simulink model "arduino_serial_sendreceive"  (R2018a)
settings: Solver=FixedStepAuto  StartTime=0.0  StopTime=inf  FixedStep=0.005  RelTol=1e-3  EnableMultiTasking=on
undefined symbols (not defined in the file or in its folder): maxPWM, minPWM
libraries: arduinolib x3, simulink x1
settings Model: SimulationMode=external  ExtModeTrigDuration=2  Creator=The MathWorks, Inc.  LastModifiedBy=adiravishankara
settings SolverCC: AutoInsertRateTranBlk=on
settings OptimizationCC: PassReuseOutputArgsThreshold=0  MaxStackSize=64
settings DebuggingCC: ParameterTunabilityLossMsg=error
settings HardwareCC: ProdBitPerPointer=32  ProdBitPerSizeT=32  ProdBitPerPtrDiffT=32  ProdLargestAtomicInteger=Long  ProdLargestAtomicFloat=Double  ProdWordSize=32  ProdHWDeviceType=ARM Compatible->ARM Cortex  UseEmbeddedCoderFeatures=off
settings SFSimCC: MATLABDynamicMemAlloc=off
settings RTWCC: SystemTargetFile=ert.tlc  HardwareBoard=Arduino Due  TLCOptions=-aInlineSetEventsForThisBaseRateFcn=TLC_FALSE -aSuppressMultiTaskScheduler=TLC_FALSE -aRateBasedStepFcn=1  TemplateMakefile=ert_default_tmf  GenerateReport=on  Toolchain=Arduino ARM  BuildConfiguration=Faster Runs  LaunchReport=on
settings CodeAppCC: ForceParamTrailComments=on  OperatorAnnotations=on
settings ERTTargetCC: ERTCustomFileBanners=off  SupportContinuousTime=on  SupportNonInlinedSFcns=on  RemoveResetFunc=off  SupportVariableSizeSignals=on  ModelStepFunctionPrototypeControlCompliant=off

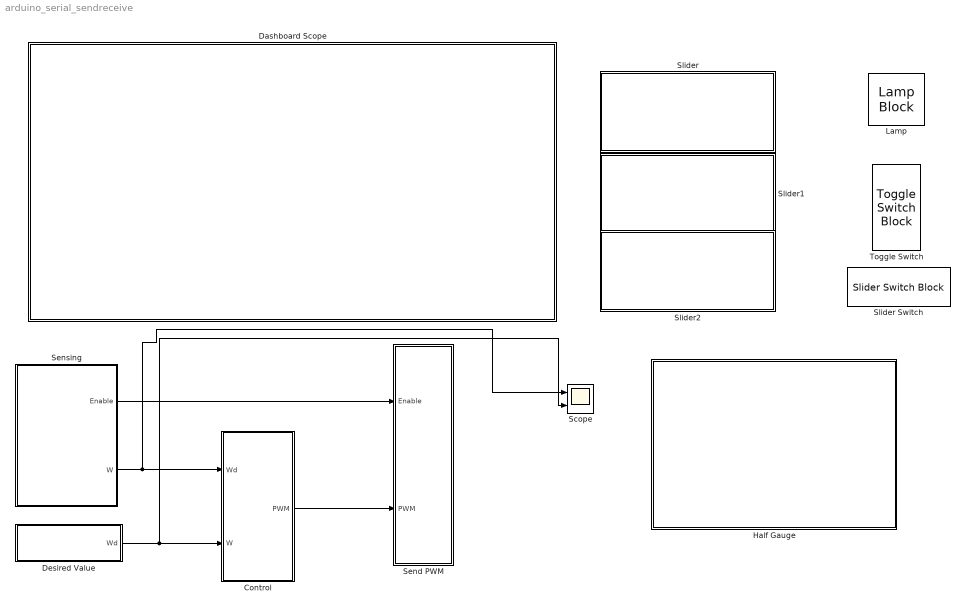
== system arduino_serial_sendreceive ==
  Control : Subsystem
  Dashboard Scope : Subsystem  DialogController=hmiCreateDDGDialog  IsWebBlock=on  mask(MWDashboardBlock){webBlockId=9cdac41f-9582-470c-8574-661c351767b2, webBlockType=sdiscope, ShowInitialText=on, HMISrcModelName=arduino_serial_sendreceive}
      mask prompts: webBlockId "WebBlock Id"; webBlockType "WebBlock Type"; HMISrcModelName "Source Model"
      mask help: SimulinkHMI:dialogs:HMIScopeDialogDesc
      mask Help: helpview([docroot '/mapfiles/simulink.map'], 'hmi_scope')
      mask Display:
      | if strcmp(get_param(bdroot(gcb),'BlockDiagramType'), 'library')
      |     image([(matlabroot) '/toolbox/simulink/hmi/icons/DashboardScope.png']);
      | end
  Desired Value : Subsystem
  Half Gauge : Subsystem  DialogController=hmiCreateDDGDialog  IsWebBlock=on  mask(MWDashboardBlock){webBlockId=e40b3037-9584-4a9a-b861-680f52ec12d3, webBlockType=semicirculargauge, ShowInLibBrowser=on, ShowInitialText=on, HMISrcModelName=arduino_serial_sendreceive}
      mask prompts: webBlockId "WebBlock Id"; webBlockType "WebBlock Type"; HMISrcModelName "Source Model"
      mask help: SimulinkHMI:dialogs:SemicircularGaugeDialogDesc
      mask Help: helpview([docroot '/mapfiles/simulink.map'], 'hmi_half_gauge')
      mask Display:
      | if strcmp(get_param(bdroot(gcb),'BlockDiagramType'), 'library')
      |     image([(matlabroot) '/toolbox/simulink/hmi/icons/SemicircularGauge.png']);
      | end
  Lamp : LampBlock  WebBlockId=101
  Scope : Scope  NumInputPorts=2
  Send PWM : Subsystem
  Sensing : Subsystem
  Slider : Subsystem  DialogController=hmiCreateDDGDialog  IsWebBlock=on  mask(MWDashboardBlock){webBlockId=dae65e69-4071-40d6-a268-0e0f4e1137e4, webBlockType=slider, ShowInLibBrowser=on, ShowInitialText=on, HMISrcModelName=arduino_serial_sendreceive}
      mask prompts: webBlockId "WebBlock Id"; webBlockType "WebBlock Type"; HMISrcModelName "Source Model"
      mask help: SimulinkHMI:dialogs:SliderDialogDesc
      mask Help: helpview([docroot '/mapfiles/simulink.map'], 'hmi_slider')
      mask Display:
      | if strcmp(get_param(bdroot(gcb),'BlockDiagramType'), 'library')
      |     image([(matlabroot) '/toolbox/simulink/hmi/icons/Slider.png']);
      | end
  Slider Switch : SliderSwitchBlock  WebBlockId=56
      settings: Values={{'Off', 'On'}, [0 1]}
  Slider1 : Subsystem  DialogController=hmiCreateDDGDialog  IsWebBlock=on  mask(MWDashboardBlock){webBlockId=011a6a40-20fb-436f-979b-6126fe8aa68b, webBlockType=slider, ShowInLibBrowser=on, ShowInitialText=on, HMISrcModelName=arduino_serial_sendreceive}
      mask prompts: webBlockId "WebBlock Id"; webBlockType "WebBlock Type"; HMISrcModelName "Source Model"
      mask help: SimulinkHMI:dialogs:SliderDialogDesc
      mask Help: helpview([docroot '/mapfiles/simulink.map'], 'hmi_slider')
      mask Display:
      | if strcmp(get_param(bdroot(gcb),'BlockDiagramType'), 'library')
      |     image([(matlabroot) '/toolbox/simulink/hmi/icons/Slider.png']);
      | end
  Slider2 : Subsystem  DialogController=hmiCreateDDGDialog  IsWebBlock=on  mask(MWDashboardBlock){webBlockId=c4424a9c-954c-4801-934e-159076550821, webBlockType=slider, ShowInLibBrowser=on, ShowInitialText=on, HMISrcModelName=arduino_serial_sendreceive}
      mask prompts: webBlockId "WebBlock Id"; webBlockType "WebBlock Type"; HMISrcModelName "Source Model"
      mask help: SimulinkHMI:dialogs:SliderDialogDesc
      mask Help: helpview([docroot '/mapfiles/simulink.map'], 'hmi_slider')
      mask Display:
      | if strcmp(get_param(bdroot(gcb),'BlockDiagramType'), 'library')
      |     image([(matlabroot) '/toolbox/simulink/hmi/icons/Slider.png']);
      | end
  Toggle Switch : ToggleSwitchBlock  WebBlockId=59
      settings: Values={{'Off', 'On'}, [0 1]}
  wires:
  Desired Value/1(Wd) -> Scope/2, Control/2(W)
  Control/1(PWM) -> Send PWM/2(PWM)
  Sensing/2(W) -> Scope/1, Control/1(Wd)
  Sensing/1(Enable) -> Send PWM/1(Enable)

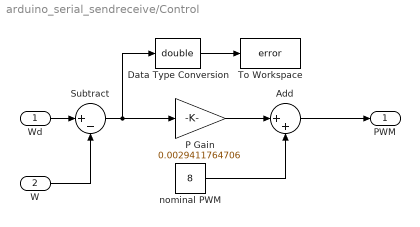
== system arduino_serial_sendreceive/Control ==
  Wd : Inport
  W : Inport  Port=2
  Add : Sum  Inputs=|++
  Data Type Conversion : DataTypeConversion  OutDataTypeStr=double
  P Gain : Gain  Gain=0.0029411764706
  Subtract : Sum  Inputs=|+-
  To Workspace : ToWorkspace  VariableName=error  SaveFormat=Structure With Time  SampleTime=-1
  nominal PWM : Constant  Value=8
  PWM : Outport
  wires:
  nominal PWM/1 -> Add/2
  Add/1 -> PWM/1
  Wd/1 -> Subtract/1
  W/1 -> Subtract/2
  P Gain/1 -> Add/1
  Data Type Conversion/1 -> To Workspace/1
  Subtract/1 -> Data Type Conversion/1, P Gain/1

== system arduino_serial_sendreceive/Dashboard Scope ==

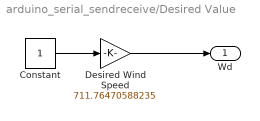
== system arduino_serial_sendreceive/Desired Value ==
  Constant : Constant
  "Desired Wind Speed " : Gain  Gain=711.76470588235
  Wd : Outport
  wires:
  Constant/1 -> "Desired Wind Speed "/1
  "Desired Wind Speed "/1 -> Wd/1

== system arduino_serial_sendreceive/Half Gauge ==

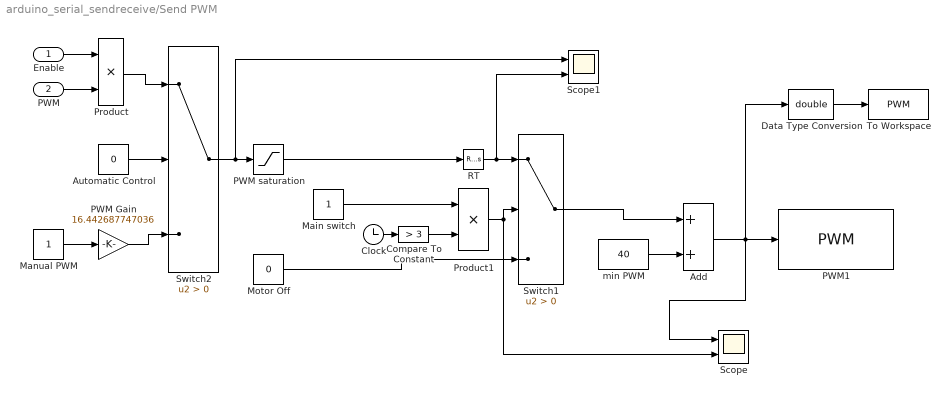
== system arduino_serial_sendreceive/Send PWM ==
  Enable : Inport
  PWM : Inport  Port=2
  Add : Sum
  Automatic Control : Constant  Value=0
  Clock : Clock
  Compare To Constant : simulink/Logic and Bit Operations/Compare To Constant  relop=>  const=3  OutDataTypeStr=boolean
  Data Type Conversion : DataTypeConversion  OutDataTypeStr=double
  Main switch : Constant
  Manual PWM : Constant
  Motor Off : Constant  Value=0
  PWM Gain : Gain  Gain=16.442687747036
  PWM saturation : Saturate  UpperLimit=maxPWM  LowerLimit=minPWM
  PWM1 : arduinolib/PWM  pinNumber=12  EnableInputFrequency=off  InitialFrequency=2000  InitialDutyCycle=0  NotificationType=None  blockPlatform=arduino
  Product : Product
  Product1 : Product
  RT : RateTransition  OutPortSampleTime=0.005
  Scope : Scope  NumInputPorts=2
  Scope1 : Scope  NumInputPorts=2
  Switch1 : Switch  Criteria=u2 > Threshold
  Switch2 : Switch  Criteria=u2 > Threshold
  To Workspace : ToWorkspace  VariableName=PWM  SaveFormat=Structure With Time  SampleTime=-1
  min PWM : Constant  Value=40
  wires:
  PWM saturation/1 -> RT/1
  Motor Off/1 -> Switch1/3
  Add/1 -> Scope/1, Data Type Conversion/1, PWM1/1
  min PWM/1 -> Add/2
  Main switch/1 -> Product1/1
  PWM/1 -> Product/2
  Automatic Control/1 -> Switch2/2
  Manual PWM/1 -> PWM Gain/1
  Switch2/1 -> Scope1/1, PWM saturation/1
  PWM Gain/1 -> Switch2/3
  Enable/1 -> Product/1
  Product/1 -> Switch2/1
  Data Type Conversion/1 -> To Workspace/1
  Switch1/1 -> Add/1
  Clock/1 -> Compare To Constant/1
  Compare To Constant/1 -> Product1/2
  Product1/1 -> Scope/2, Switch1/2
  RT/1 -> Scope1/2, Switch1/1

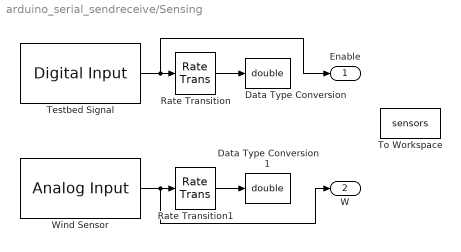
== system arduino_serial_sendreceive/Sensing ==
  Data Type Conversion : DataTypeConversion  OutDataTypeStr=double
  Data Type Conversion1 : DataTypeConversion  OutDataTypeStr=double
  Rate Transition : RateTransition
  Rate Transition1 : RateTransition
  "Testbed Signal " : arduinolib/Digital Input  pinNumber=3  sampleTime=0.1  blockPlatform=arduino
      settings: SourceProductName=Simulink Support Package for Arduino Hardware
  To Workspace : ToWorkspace  VariableName=sensors  SaveFormat=Structure With Time  SampleTime=-1
  Wind Sensor : arduinolib/Analog Input  pinNumber=2  ReadResultsOnly=off  ConversionTriggerSource=Software  ExternalTriggerType=uint32(0)  OutputDataType=uint16  EnableConversionCompleteNotify=off  EnableOuputStatus=off  SampleTime=0.01  blockPlatform=arduino
  Enable : Outport
  W : Outport  Port=2
  wires:
  Wind Sensor/1 -> W/1, Rate Transition1/1
  "Testbed Signal "/1 -> Enable/1, Rate Transition/1
  Rate Transition/1 -> Data Type Conversion/1
  Rate Transition1/1 -> Data Type Conversion1/1

== system arduino_serial_sendreceive/Slider ==

== system arduino_serial_sendreceive/Slider1 ==

== system arduino_serial_sendreceive/Slider2 ==
